simulink model "c10mcaputo"  (Simulink 7.1)
settings: Solver=ode45  StartTime=0.001  StopTime=1  RelTol=1e-10
settings Model: Creator=toshiba  LastModifiedBy=Administrator
settings OptimizationCC: InitFltsAndDblsToZero=off
settings DebuggingCC: StrictBusMsg=ErrorLevel1

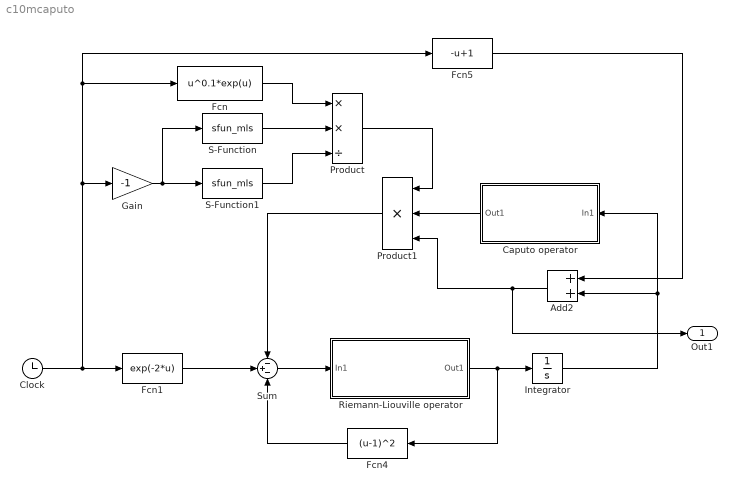
== system c10mcaputo ==
  Add2 : Sum  Orientation=left
  Caputo operator : Subsystem  Orientation=left  mask{gam=0.555, ww=[0.001 1000], n=9, a=[-1 1]}
      mask prompts: gam "D"; ww "F"; n "A"; a "C"
      mask init:
      | wb=ww(1); wh=ww(2);G=ousta_fod(gam,n,wb,wh); G1=tf(G);
      | num=G1.num{1}; den=G1.den{1}; T=1/wh;
      | set_param('c10mcaputo/Caputo operator/Fcn','Expr',char(poly2caputo(a,gam)));
      | str='Fractional\n';
      | if isnumeric(gam)
      | if gam>0, str=[str, 'Der s^' num2str(gam) ];
      | else, str=[str, 'Int s^{' num2str(gam) '}']; end
      | else, str=[str, 'Der s^gam']; end
      mask Display: disp(str)
  Clock : Clock
      settings: Decimation=10
  Fcn : Fcn  Expr=u^0.1*exp(u)
  Fcn1 : Fcn  Expr=exp(-2*u)
  Fcn4 : Fcn  Orientation=left  Expr=(u-1)^2
  Fcn5 : Fcn  Expr=-u+1
  Gain : Gain  Gain=-1
  Integrator : Integrator
  Product : Product  Inputs=**/  RndMeth=Zero
  Product1 : Product  Orientation=left  Inputs=3  RndMeth=Zero
  Riemann-Liouville operator : Subsystem  mask{gam=-0.455, ww=[0.001  1000], n=9}
      mask prompts: gam "D"; ww "F"; n "A"
      mask init:
      | wb=ww(1); wh=ww(2);G=ousta_fod(gam,n,wb,wh);
      | G1=tf(G)
      | num=G1.num{1}; den=G1.den{1}; T=1/wh;
      | str='Fractional\n';
      | if isnumeric(gam)
      | if gam>0, str=[str, 'Der s^' num2str(gam) ];
      | else, str=[str, 'Int s^{' num2str(gam) '}']; end
      | else, str=[str, 'Der s^gam']; end
      mask Display: disp(str)
  S-Function : S-Function  FunctionName=sfun_mls  Parameters=1.545  EnableBusSupport=off
  S-Function1 : S-Function  FunctionName=sfun_mls  Parameters=1.445  EnableBusSupport=off
  Sum : Sum  Inputs=-+-
  Out1 : Outport
  wires:
  Clock/1 -> Fcn1/1, Gain/1, Fcn/1, Fcn5/1
  Gain/1 -> S-Function/1, S-Function1/1
  Fcn/1 -> Product/1
  S-Function/1 -> Product/2
  S-Function1/1 -> Product/3
  Fcn1/1 -> Sum/2
  Product1/1 -> Sum/1
  Product/1 -> Product1/1
  Fcn4/1 -> Sum/3
  Integrator/1 -> Add2/2, Caputo operator/1(In1)
  Add2/1 -> Product1/3, Out1/1
  Fcn5/1 -> Add2/1
  Sum/1 -> Riemann-Liouville operator/1(In1)
  Riemann-Liouville operator/1(Out1) -> Integrator/1, Fcn4/1
  Caputo operator/1(Out1) -> Product1/2

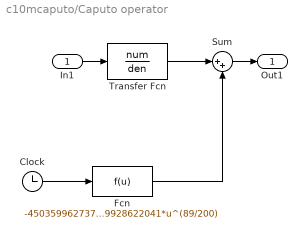
== system c10mcaputo/Caputo operator ==
  In1 : Inport
  Clock : Clock
      settings: Decimation=10
  Fcn : Fcn  Expr=-450359962737049600/398893879928622041*u^(89/200)
  Sum : Sum  Inputs=|++
  Transfer Fcn : TransferFcn  Numerator=num  Denominator=den
  Out1 : Outport
  wires:
  Clock/1 -> Fcn/1
  Transfer Fcn/1 -> Sum/1
  Sum/1 -> Out1/1
  In1/1 -> Transfer Fcn/1
  Fcn/1 -> Sum/2

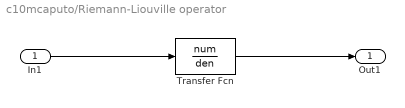
== system c10mcaputo/Riemann-Liouville operator ==
  In1 : Inport
  Transfer Fcn : TransferFcn  Numerator=num  Denominator=den
  Out1 : Outport
  wires:
  In1/1 -> Transfer Fcn/1
  Transfer Fcn/1 -> Out1/1
